simulink model "PubIfDecisionTOS_MDL"  (R2020b)
settings: configuration reference "DspaceConfig" (kept outside this file)
PostLoadFcn:
  | if any(exist('dsrtsu_mdlpostloadfcn', 'file') ~= 0), dsrtsu_mdlpostloadfcn('Execute', bdroot); end
InitFcn:
  | , if any(exist('dsmpb_private', 'file') ~= 0), dsmpb_private('dsmpb_mdlclblib', 'Init', bdroot); end,
undefined symbols (not defined in the file or in its folder): C_TOS_ACCEgoRAxletoFbumplength_m, C_TOS_ACCTargetFront_Flag, C_TOS_AEBJAPedObjDxThre_Val, C_TOS_AEBJAPedObjDyThre_Val, C_TOS_AEBJATargetSize_Val, C_TOS_AEBJAVehObjDxThre_Val, C_TOS_AEBJAVehObjDyThre_Val, C_TOS_AEBJuncPedTargetSize_Val, C_TOS_AEBLatObjDxThre_Val, C_TOS_AEBLatPedDyThre_Val, C_TOS_AEBLatTargetSize_Val, C_TOS_AEBLongTargetInEgoFront_Flag, C_TOS_axAbsGround_Parameter, C_TOS_CameraConfirmedFlag, C_TOS_CNsubjWidth, C_TOS_CurrentLaneCoreMinWidth_Val, C_TOS_CutInProb_Val_Zero, C_TOS_CutOutProb_Val_Zero, C_TOS_D2R_Val, C_TOS_DefaultValueObjectToCenterLine_dy, C_TOS_EgoCarWidth_Val, C_TOS_EgoDxRefPoint_m, C_TOS_EgoRAxletoFbumplength_m, C_TOS_HalfWidthVehicle_Con, C_TOS_HWA_CurrentLaneFlag, C_TOS_HWA_LeftLaneFlag, C_TOS_HWA_MovingDir_Vaild, C_TOS_HWA_MovState_Vaild, C_TOS_HWA_RightLaneFlag, C_TOS_LaneLineCourseErrorFront, C_TOS_LaneLineCourseErrorRear, C_TOS_MotorbikeDefaultWidth_m, C_TOS_NumberOfEffectiveTargets, C_TOS_Obj_Age_Val, C_TOS_Objdx_Constraint_Val, C_TOS_ObjectDefaultWidth_m, C_TOS_ObjInCurrentLane_Val, C_TOS_ObjInCurrentLaneValid, C_TOS_ObjInLeftLaneValid, C_TOS_ObjInRightLaneValid, C_TOS_ObjNotInCurrentLane_Val, C_TOS_ObjNotREElementType, C_TOS_ObjPredictDis_dy_ConstantVal_Zeros, C_TOS_ObjToCenterLine_ConstantVal_Zeros, C_TOS_OFMObjIDInvilad_Val, C_TOS_PIL_LatDisCons_Val_zero, C_TOS_PIL_ObjectCutInFlag_b, C_TOS_PIL_ObjectCutOutFlag_b, C_TOS_PIL_ObjLaneProb_al_Val, C_TOS_PP_ObjFusType_FC_Confirm_b, C_TOS_PP_ObjFusType_FC_FR_Confirm_b, C_TOS_PP_ObjFusType_FR_Confirm_b, C_TOS_RE_80BoolDefault_Val, C_TOS_RE_80Single181Default_Val, C_TOS_RE_80Single255Default_Val, C_TOS_RE_80Uint8Default_Val, C_TOS_RE_D2R, C_TOS_RE_D_180_Val, C_TOS_RE_InvalidObjectID_Val, C_TOS_RE_InvalidTargetChainDir_Val ... (+142)
libraries: simulink x1650, TOS_LIB x361, canfdmsglib x14
(part 4 of 69)

== system PubIfDecisionTOS_MDL/TOS_20201112/TOS_2012080320/Subsystem3 ==
  TOS_ELK : Inport
  TOS_LC : Inport  Port=2
  TOS_LCKIE : Inport  Port=3
  Bus Selector : BusSelector  OutputSignals=Object_DX,Object_DY,Object_Fus_Type,Object_Type,Object_VX
  Bus Selector1 : BusSelector  OutputSignals=Object_DX,Object_DY,Object_ExistProb,Object_Fus_Type,Object_ID,Object_Type
  Bus Selector2 : BusSelector  OutputSignals=CurrentLane_Prob,LeftLane_Prob,Object_ExistProb,Object_Fus_Type,Object_ID,Object_MovingState,Object_ObstacleProb,Object_Orientation,Object_Type,RightLane_Prob
  Bus Selector3 : BusSelector  OutputSignals=ObjectIn_Lane,Object_DX,Object_DY,Object_VX
  Bus Selector4 : BusSelector  OutputSignals=CurrentLane_Prob,LeftLane_Prob,ObjectIn_Lane,Object_ExistProb,Object_ID,Object_ObstacleProb
  Bus Selector5 : BusSelector  OutputSignals=CurrentLane_Prob,LeftLane_Prob,ObjectIn_Lane,Object_VX,RightLane_Prob
  CAN FD Pack : canfdmsglib/CAN FD Pack  CANdbFile=F:\InternalData03_ACC_AEBLog_ELK_LC_LCKie_20200927.dbc  MsgList=(none)  MsgName=TOS_ELK_1  ProtocolMode=CAN FD  MsgIDType=Standard (11-bit identifier)  MsgIdentifier=515  MsgLength=64  Remote=off  BRSSwitch=off  ApplyMinMax=off  SignalInfo={'{'ELK_CurrentLane_Prob_01','289','7','BE','unsigned','Standard','0','0.01','0','0','1.27';'ELK_CurrentLane_Prob_02','65','7','BE','unsigned','Standard','0','0.01','0','0','1.27';'ELK_CurrentLane_Prob_03','73','7','BE','unsigned','Standard','0','0.01','0','0','1.27';'ELK_CurrentLane_Prob_04','113','7','BE','unsigned','Standard','0','0.01','0','0','1.27';'ELK_CurrentLane_Prob_05','121','7','BE','unsigned','Standard','0','0.01','0','0','1.27';'ELK_CurrentLane_Prob_06','193','7','BE','unsigned','Standard','0','0.01','0','0','1.27';'ELK_CurrentLane_Prob_07','201','7','BE','unsigned','Standard','0','0.01','0','0','1.27';'ELK_CurrentLane_Prob_08','241','7','BE','unsigned','Standard','0','0.01','0','0','1.27';'ELK_LeftLane_Prob_01','281','7','BE','unsigned','Standard','0','0.01','0','0','1.27';'ELK_LeftLane_Prob_02','297','7','BE','unsigned','Standard','0','0.01','0','0','1.27';'ELK_LeftLane_Prob_03','305','7','BE','unsigned','Standard','0','0.01','0','0','1.27';'ELK_LeftLane_Prob_04','313','7','BE','unsigned','Standard','0','0.01','0','0','1.27';'ELK_LeftLane_Prob_05','321','7','BE','unsigned','Standard','0','0.01','0','0','1.27';'ELK_LeftLane_Prob_06','329','7','BE','unsigned','Standard','0','0.01','0','0','1.27';'ELK_LeftLane_Prob_07','337','7','BE','unsigned','Standard','0','0.01','0','0','1.27';'ELK_LeftLane_Prob_08','345','7','BE','unsigned','Standard','0','0.01','0','0','1.27';'ELK_Object_ExistProb_01','369','7','BE','unsigned','Standard','0','0.007875','0','0','1.0001';'ELK_Object_ExistProb_02','377','7','BE','unsigned','Standard','0','0.007875','0','0','1.0001';'ELK_Object_ExistProb_03','385','7','BE','unsigned','Standard','0','0.007875','0','0','1.0001';'ELK_Object_ExistProb_04','393','7','BE','unsigned','Standard','0','0.007875','0','0','1.0001';'ELK_Object_ExistProb_05','401','7','BE','unsigned','Standard','0','0.007875','0','0','1.0001';'ELK_Object_ExistProb_06','409','7','BE','unsigned','Standard','0','0.007875','0','0','1.0001';'ELK_Object_ExistProb_07','417','7','BE','unsigned','Standard','0','0.007875','0','0','1.0001';'ELK_Object_ExistProb_08','425','7','BE','unsigned','Standard','0','0.007875','0','0','1.0001';'ELK_Object_Fus_Type_01','452','4','BE','unsigned','Standard','0','1','0','0','15';'ELK_Object_Fus_Type_02','448','4','BE','unsigned','Standard','0','1','0','0','15';'ELK_Object_Fus_Type_03','460','4','BE','unsigned','Standard','0','1','0','0','15';'ELK_Object_Fus_Type_04','456','4','BE','unsigned','Standard','0','1','0','0','15';'ELK_Object_Fus_Type_05','468','4','BE','unsigned','Standard','0','1','0','0','15';'ELK_Object_Fus_Type_06','464','4','BE','unsigned','Standard','0','1','0','0','15';'ELK_Object_Fus_Type_07','476','4','BE','unsigned','Standard','0','1','0','0','15';'ELK_Object_Fus_Type_08','472','4','BE','unsigned','Standard','0','1','0','0','15';'ELK_Object_ID_01','1','7','BE','unsigned','Standard','0','1','0','0','127';'ELK_Object_ID_02','9','7','BE','unsigned','Standard','0','1','0','0','127';'ELK_Object_ID_03','17','7','BE','unsigned','Standard','0','1','0','0','127';'ELK_Object_ID_04','25','7','BE','unsigned','Standard','0','1','0','0','127';'ELK_Object_ID_05','33','7','BE','unsigned','Standard','0','1','0','0','127';'ELK_Object_ID_06','41','7','BE','unsigned','Standard','0','1','0','0','127';'ELK_Object_ID_07','49','7','BE','unsigned','Standard','0','1','0','0','127';'ELK_Object_ID_08','57','7','BE','unsigned','Standard','0','1','0','0','127';'ELK_Object_MovingState_01','85','3','BE','unsigned','Standard','0','1','0','0','7';'ELK_Object_MovingState_02','82','3','BE','unsigned','Standard','0','1','0','0','7';'ELK_Object_MovingState_03','93','3','BE','unsigned','Standard','0','1','0','0','7';'ELK_Object_MovingState_04','90','3','BE','unsigned','Standard','0','1','0','0','7';'ELK_Object_MovingState_05','101','3','BE','unsigned','Standard','0','1','0','0','7';'ELK_Object_MovingState_06','98','3','BE','unsigned','Standard','0','1','0','0','7';'ELK_Object_MovingState_07','109','3','BE','unsigned','Standard','0','1','0','0','7';'ELK_Object_MovingState_08','106','3','BE','unsigned','Standard','0','1','0','0','7';'ELK_Object_ObstacleProb_01','129','7','BE','unsigned','Standard','0','0.007875','0','0','1.0001';'ELK_Object_ObstacleProb_02','137','7','BE','unsigned','Standard','0','0.007875','0','0','1.0001';'ELK_Object_ObstacleProb_03','145','7','BE','unsigned','Standard','0','0.007875','0','0','1.0001';'ELK_Object_ObstacleProb_04','153','7','BE','unsigned','Standard','0','0.007875','0','0','1.0001';'ELK_Object_ObstacleProb_05','161','7','BE','unsigned','Standard','0','0.007875','0','0','1.0001';'ELK_Object_ObstacleProb_06','169','7','BE','unsigned','Standard','0','0.007875','0','0','1.0001';'ELK_Object_ObstacleProb_07','177','7','BE','unsigned','Standard','0','0.007875','0','0','1.0001';'ELK_Object_ObstacleProb_08','185','7','BE','unsigned','Standard','0','0.007875','0','0','1.0001';'ELK_Object_Orientation_01','212','4','BE','unsigned','Standard','0','1','0','0','15';'ELK_Object_Orientation_02','208','4','BE','unsigned','Standard','0','1','0','0','15';'ELK_Object_Orientation_03','220','4','BE','unsigned','Standard','0','1','0','0','15';'ELK_Object_Orientation_04','216','4','BE','unsigned','Standard','0','1','0','0','15';'ELK_Object_Orientation_05','228','4','BE','unsigned','Standard','0','1','0','0','15';'ELK_Object_Orientation_06','224','4','BE','unsigned','Standard','0','1','0','0','15';'ELK_Object_Orientation_07','236','4','BE','unsigned','Standard','0','1','0','0','15';'ELK_Object_Orientation_08','232','4','BE','unsigned','Standard','0','1','0','0','15';'ELK_Object_Type_01','252','4','BE','unsigned','Standard','0','1','0','0','15';'ELK_Object_Type_02','248','4','BE','unsigned','Standard','0','1','0','0','15';'ELK_Object_Type_03','260','4','BE','unsigned','Standard','0','1','0','0','15';'ELK_Object_Type_04','256','4','BE','unsigned','Standard','0','1','0','0','15';'ELK_Object_Type_05','268','4','BE','unsigned','Standard','0','1','0','0','15';'ELK_Object_Type_06','264','4','BE','unsigned','Standard','0','1','0','0','15';'ELK_Object_Type_07','276','4','BE','unsigned','Standard','0','1','0','0','15';'ELK_Object_Type_08','272','4','BE','unsigned','Standard','0','1','0','0','15';'ELK_RightLane_Prob_01','353','7','BE','unsigned','Standard','0','0.01','0','0','1.27';'ELK_RightLane_Prob_02','361','7','BE','unsigned','Standard','0','0.01','0','0','1.27';'ELK_RightLane_Prob_03','433','7','BE','unsigned','Standard','0','0.01','0','0','1.27';'ELK_RightLane_Prob_04','441','7','BE','unsigned','Standard','0','0.01','0','0','1.27';'ELK_RightLane_Prob_05','481','7','BE','unsigned','Standard','0','0.01','0','0','1.27';'ELK_RightLane_Prob_06','489','7','BE','unsigned','Standard','0','0.01','0','0','1.27';'ELK_RightLane_Prob_07','497','7','BE','unsigned','Standard','0','0.01','0','0','1.27'}
      settings: SourceProductBaseCode=VN  DataFormat=CANdb specified signals
  CAN FD Pack1 : canfdmsglib/CAN FD Pack  CANdbFile=F:\InternalData03_ACC_AEBLog_ELK_LC_LCKie_20200927.dbc  MsgList=(none)  MsgName=TOS_ELK_2  ProtocolMode=CAN FD  MsgIDType=Standard (11-bit identifier)  MsgIdentifier=516  MsgLength=64  Remote=off  BRSSwitch=off  ApplyMinMax=off  SignalInfo={'{'ELK_ObjectIn_Lane_01','132','4','BE','unsigned','Standard','0','1','0','0','15';'ELK_ObjectIn_Lane_02','128','4','BE','unsigned','Standard','0','1','0','0','15';'ELK_ObjectIn_Lane_03','140','4','BE','unsigned','Standard','0','1','0','0','15';'ELK_ObjectIn_Lane_04','136','4','BE','unsigned','Standard','0','1','0','0','15';'ELK_ObjectIn_Lane_05','148','4','BE','unsigned','Standard','0','1','0','0','15';'ELK_ObjectIn_Lane_06','144','4','BE','unsigned','Standard','0','1','0','0','15';'ELK_ObjectIn_Lane_07','156','4','BE','unsigned','Standard','0','1','0','0','15';'ELK_ObjectIn_Lane_08','152','4','BE','unsigned','Standard','0','1','0','0','15';'ELK_Object_DX_01','8','16','BE','signed','Standard','0','0.01','0','-327.68','327.67';'ELK_Object_DX_02','24','16','BE','signed','Standard','0','0.01','0','-327.68','327.67';'ELK_Object_DX_03','40','16','BE','signed','Standard','0','0.01','0','-327.68','327.67';'ELK_Object_DX_04','56','16','BE','signed','Standard','0','0.01','0','-327.68','327.67';'ELK_Object_DX_05','72','16','BE','signed','Standard','0','0.01','0','-327.68','327.67';'ELK_Object_DX_06','88','16','BE','signed','Standard','0','0.01','0','-327.68','327.67';'ELK_Object_DX_07','104','16','BE','signed','Standard','0','0.01','0','-327.68','327.67';'ELK_Object_DX_08','120','16','BE','signed','Standard','0','0.01','0','-327.68','327.67';'ELK_Object_DY_01','168','16','BE','signed','Standard','0','0.01','0','-327.68','327.67';'ELK_Object_DY_02','184','16','BE','signed','Standard','0','0.01','0','-327.68','327.67';'ELK_Object_DY_03','200','16','BE','signed','Standard','0','0.01','0','-327.68','327.67';'ELK_Object_DY_04','216','16','BE','signed','Standard','0','0.01','0','-327.68','327.67';'ELK_Object_DY_05','232','16','BE','signed','Standard','0','0.01','0','-327.68','327.67';'ELK_Object_DY_06','248','16','BE','signed','Standard','0','0.01','0','-327.68','327.67';'ELK_Object_DY_07','264','16','BE','signed','Standard','0','0.01','0','-327.68','327.67';'ELK_Object_DY_08','280','16','BE','signed','Standard','0','0.01','0','-327.68','327.67';'ELK_Object_VX_01','332','12','BE','signed','Standard','0','0.1','0','-204.8','204.7';'ELK_Object_VX_02','348','12','BE','signed','Standard','0','0.1','0','-204.8','204.7';'ELK_Object_VX_03','364','12','BE','signed','Standard','0','0.1','0','-204.8','204.7';'ELK_Object_VX_04','380','12','BE','signed','Standard','0','0.1','0','-204.8','204.7';'ELK_Object_VX_05','396','12','BE','signed','Standard','0','0.1','0','-204.8','204.7';'ELK_Object_VX_06','412','12','BE','signed','Standard','0','0.1','0','-204.8','204.7';'ELK_Object_VX_07','428','12','BE','signed','Standard','0','0.1','0','-204.8','204.7'}
      settings: SourceProductBaseCode=VN  DataFormat=CANdb specified signals
  CAN FD Pack2 : canfdmsglib/CAN FD Pack  CANdbFile=F:\InternalData03_ACC_AEBLog_ELK_LC_LCKie_20200927.dbc  MsgList=(none)  MsgName=TOS_LC_1  ProtocolMode=CAN FD  MsgIDType=Standard (11-bit identifier)  MsgIdentifier=519  MsgLength=64  Remote=off  BRSSwitch=off  ApplyMinMax=off  SignalInfo={'{'LC_Object_DX_01','12','12','BE','signed','Standard','0','0.1','0','-204.8','204.7';'LC_Object_DX_02','28','12','BE','signed','Standard','0','0.1','0','-204.8','204.7';'LC_Object_DX_03','44','12','BE','signed','Standard','0','0.1','0','-204.8','204.7';'LC_Object_DX_04','60','12','BE','signed','Standard','0','0.1','0','-204.8','204.7';'LC_Object_DX_05','76','12','BE','signed','Standard','0','0.1','0','-204.8','204.7';'LC_Object_DX_06','92','12','BE','signed','Standard','0','0.1','0','-204.8','204.7';'LC_Object_DX_07','108','12','BE','signed','Standard','0','0.1','0','-204.8','204.7';'LC_Object_DX_08','124','12','BE','signed','Standard','0','0.1','0','-204.8','204.7';'LC_Object_DX_09','140','12','BE','signed','Standard','0','0.1','0','-204.8','204.7';'LC_Object_DX_10','156','12','BE','signed','Standard','0','0.1','0','-204.8','204.7';'LC_Object_DX_11','172','12','BE','signed','Standard','0','0.1','0','-204.8','204.7';'LC_Object_DY_01','188','12','BE','signed','Standard','0','0.1','0','-204.8','204.7';'LC_Object_DY_02','204','12','BE','signed','Standard','0','0.1','0','-204.8','204.7';'LC_Object_DY_03','220','12','BE','signed','Standard','0','0.1','0','-204.8','204.7';'LC_Object_DY_04','236','12','BE','signed','Standard','0','0.1','0','-204.8','204.7';'LC_Object_DY_05','252','12','BE','signed','Standard','0','0.1','0','-204.8','204.7';'LC_Object_DY_06','268','12','BE','signed','Standard','0','0.1','0','-204.8','204.7';'LC_Object_DY_07','284','12','BE','signed','Standard','0','0.1','0','-204.8','204.7';'LC_Object_DY_08','300','12','BE','signed','Standard','0','0.1','0','-204.8','204.7';'LC_Object_DY_09','316','12','BE','signed','Standard','0','0.1','0','-204.8','204.7';'LC_Object_DY_10','332','12','BE','signed','Standard','0','0.1','0','-204.8','204.7';'LC_Object_DY_11','348','12','BE','signed','Standard','0','0.1','0','-204.8','204.7';'LC_Object_Fus_Type_01','8','4','BE','unsigned','Standard','0','1','0','0','15';'LC_Object_Fus_Type_02','24','4','BE','unsigned','Standard','0','1','0','0','15';'LC_Object_Fus_Type_03','40','4','BE','unsigned','Standard','0','1','0','0','15';'LC_Object_Fus_Type_04','56','4','BE','unsigned','Standard','0','1','0','0','15';'LC_Object_Fus_Type_05','72','4','BE','unsigned','Standard','0','1','0','0','15';'LC_Object_Fus_Type_06','88','4','BE','unsigned','Standard','0','1','0','0','15';'LC_Object_Fus_Type_07','104','4','BE','unsigned','Standard','0','1','0','0','15';'LC_Object_Fus_Type_08','120','4','BE','unsigned','Standard','0','1','0','0','15';'LC_Object_Fus_Type_09','136','4','BE','unsigned','Standard','0','1','0','0','15';'LC_Object_Fus_Type_10','152','4','BE','unsigned','Standard','0','1','0','0','15';'LC_Object_Fus_Type_11','168','4','BE','unsigned','Standard','0','1','0','0','15';'LC_Object_Type_01','184','4','BE','unsigned','Standard','0','1','0','0','15';'LC_Object_Type_02','200','4','BE','unsigned','Standard','0','1','0','0','15';'LC_Object_Type_03','216','4','BE','unsigned','Standard','0','1','0','0','15';'LC_Object_Type_04','232','4','BE','unsigned','Standard','0','1','0','0','15';'LC_Object_Type_05','248','4','BE','unsigned','Standard','0','1','0','0','15';'LC_Object_Type_06','264','4','BE','unsigned','Standard','0','1','0','0','15';'LC_Object_Type_07','280','4','BE','unsigned','Standard','0','1','0','0','15';'LC_Object_Type_08','296','4','BE','unsigned','Standard','0','1','0','0','15';'LC_Object_Type_09','312','4','BE','unsigned','Standard','0','1','0','0','15';'LC_Object_Type_10','328','4','BE','unsigned','Standard','0','1','0','0','15';'LC_Object_Type_11','344','4','BE','unsigned','Standard','0','1','0','0','15';'LC_Object_VX_01','384','12','BE','signed','Standard','0','0.1','0','-204.8','204.7';'LC_Object_VX_02','404','12','BE','signed','Standard','0','0.1','0','-204.8','204.7';'LC_Object_VX_03','408','12','BE','signed','Standard','0','0.1','0','-204.8','204.7';'LC_Object_VX_04','428','12','BE','signed','Standard','0','0.1','0','-204.8','204.7';'LC_Object_VX_05','432','12','BE','signed','Standard','0','0.1','0','-204.8','204.7';'LC_Object_VX_06','452','12','BE','signed','Standard','0','0.1','0','-204.8','204.7';'LC_Object_VX_07','456','12','BE','signed','Standard','0','0.1','0','-204.8','204.7';'LC_Object_VX_08','476','12','BE','signed','Standard','0','0.1','0','-204.8','204.7';'LC_Object_VX_09','480','12','BE','signed','Standard','0','0.1','0','-204.8','204.7';'LC_Object_VX_10','500','12','BE','signed','Standard','0','0.1','0','-204.8','204.7'}
      settings: SourceProductBaseCode=VN  DataFormat=CANdb specified signals
  CAN FD Pack3 : canfdmsglib/CAN FD Pack  CANdbFile=F:\InternalData03_ACC_AEBLog_ELK_LC_LCKie_20200927.dbc  MsgList=(none)  MsgName=TOS_LC_2  ProtocolMode=CAN FD  MsgIDType=Standard (11-bit identifier)  MsgIdentifier=520  MsgLength=64  Remote=off  BRSSwitch=off  ApplyMinMax=off  SignalInfo={'{'LC_CurrentLane_Prob_01','265','7','BE','unsigned','Standard','0','0.01','0','0','1.27';'LC_CurrentLane_Prob_02','273','7','BE','unsigned','Standard','0','0.01','0','0','1.27';'LC_CurrentLane_Prob_03','281','7','BE','unsigned','Standard','0','0.01','0','0','1.27';'LC_CurrentLane_Prob_04','289','7','BE','unsigned','Standard','0','0.01','0','0','1.27';'LC_CurrentLane_Prob_05','297','7','BE','unsigned','Standard','0','0.01','0','0','1.27';'LC_CurrentLane_Prob_06','305','7','BE','unsigned','Standard','0','0.01','0','0','1.27';'LC_CurrentLane_Prob_07','313','7','BE','unsigned','Standard','0','0.01','0','0','1.27';'LC_CurrentLane_Prob_08','321','7','BE','unsigned','Standard','0','0.01','0','0','1.27';'LC_CurrentLane_Prob_09','329','7','BE','unsigned','Standard','0','0.01','0','0','1.27';'LC_CurrentLane_Prob_10','337','7','BE','unsigned','Standard','0','0.01','0','0','1.27';'LC_CurrentLane_Prob_11','345','7','BE','unsigned','Standard','0','0.01','0','0','1.27';'LC_LeftLane_Prob_01','353','7','BE','unsigned','Standard','0','0.01','0','0','1.27';'LC_LeftLane_Prob_02','361','7','BE','unsigned','Standard','0','0.01','0','0','1.27';'LC_LeftLane_Prob_03','369','7','BE','unsigned','Standard','0','0.01','0','0','1.27';'LC_LeftLane_Prob_04','377','7','BE','unsigned','Standard','0','0.01','0','0','1.27';'LC_LeftLane_Prob_05','385','7','BE','unsigned','Standard','0','0.01','0','0','1.27';'LC_LeftLane_Prob_06','393','7','BE','unsigned','Standard','0','0.01','0','0','1.27';'LC_LeftLane_Prob_07','401','7','BE','unsigned','Standard','0','0.01','0','0','1.27';'LC_LeftLane_Prob_08','409','7','BE','unsigned','Standard','0','0.01','0','0','1.27';'LC_LeftLane_Prob_09','417','7','BE','unsigned','Standard','0','0.01','0','0','1.27';'LC_LeftLane_Prob_10','425','7','BE','unsigned','Standard','0','0.01','0','0','1.27';'LC_LeftLane_Prob_11','433','7','BE','unsigned','Standard','0','0.01','0','0','1.27';'LC_ObjectIn_Lane_01','444','4','BE','unsigned','Standard','0','1','0','0','15';'LC_ObjectIn_Lane_02','440','4','BE','unsigned','Standard','0','1','0','0','15';'LC_ObjectIn_Lane_03','452','4','BE','unsigned','Standard','0','1','0','0','15';'LC_ObjectIn_Lane_04','448','4','BE','unsigned','Standard','0','1','0','0','15';'LC_ObjectIn_Lane_05','460','4','BE','unsigned','Standard','0','1','0','0','15';'LC_ObjectIn_Lane_06','456','4','BE','unsigned','Standard','0','1','0','0','15';'LC_ObjectIn_Lane_07','468','4','BE','unsigned','Standard','0','1','0','0','15';'LC_ObjectIn_Lane_08','464','4','BE','unsigned','Standard','0','1','0','0','15';'LC_ObjectIn_Lane_09','476','4','BE','unsigned','Standard','0','1','0','0','15';'LC_ObjectIn_Lane_10','472','4','BE','unsigned','Standard','0','1','0','0','15';'LC_ObjectIn_Lane_11','484','4','BE','unsigned','Standard','0','1','0','0','15';'LC_Object_ExistProb_01','1','7','BE','unsigned','Standard','0','0.007875','0','0','1.0001';'LC_Object_ExistProb_02','9','7','BE','unsigned','Standard','0','0.007875','0','0','1.0001';'LC_Object_ExistProb_03','17','7','BE','unsigned','Standard','0','0.007875','0','0','1.0001';'LC_Object_ExistProb_04','25','7','BE','unsigned','Standard','0','0.007875','0','0','1.0001';'LC_Object_ExistProb_05','33','7','BE','unsigned','Standard','0','0.007875','0','0','1.0001';'LC_Object_ExistProb_06','41','7','BE','unsigned','Standard','0','0.007875','0','0','1.0001';'LC_Object_ExistProb_07','49','7','BE','unsigned','Standard','0','0.007875','0','0','1.0001';'LC_Object_ExistProb_08','57','7','BE','unsigned','Standard','0','0.007875','0','0','1.0001';'LC_Object_ExistProb_09','65','7','BE','unsigned','Standard','0','0.007875','0','0','1.0001';'LC_Object_ExistProb_10','73','7','BE','unsigned','Standard','0','0.007875','0','0','1.0001';'LC_Object_ExistProb_11','81','7','BE','unsigned','Standard','0','0.007875','0','0','1.0001';'LC_Object_ID_01','89','7','BE','unsigned','Standard','0','1','0','0','127';'LC_Object_ID_02','97','7','BE','unsigned','Standard','0','1','0','0','127';'LC_Object_ID_03','105','7','BE','unsigned','Standard','0','1','0','0','127';'LC_Object_ID_04','113','7','BE','unsigned','Standard','0','1','0','0','127';'LC_Object_ID_05','121','7','BE','unsigned','Standard','0','1','0','0','127';'LC_Object_ID_06','129','7','BE','unsigned','Standard','0','1','0','0','127';'LC_Object_ID_07','137','7','BE','unsigned','Standard','0','1','0','0','127';'LC_Object_ID_08','145','7','BE','unsigned','Standard','0','1','0','0','127';'LC_Object_ID_09','153','7','BE','unsigned','Standard','0','1','0','0','127';'LC_Object_ID_10','161','7','BE','unsigned','Standard','0','1','0','0','127';'LC_Object_ID_11','169','7','BE','unsigned','Standard','0','1','0','0','127';'LC_Object_ObstacleProb_01','177','7','BE','unsigned','Standard','0','0.007875','0','0','1.0001';'LC_Object_ObstacleProb_02','185','7','BE','unsigned','Standard','0','0.007875','0','0','1.0001';'LC_Object_ObstacleProb_03','193','7','BE','unsigned','Standard','0','0.007875','0','0','1.0001';'LC_Object_ObstacleProb_04','201','7','BE','unsigned','Standard','0','0.007875','0','0','1.0001';'LC_Object_ObstacleProb_05','209','7','BE','unsigned','Standard','0','0.007875','0','0','1.0001';'LC_Object_ObstacleProb_06','217','7','BE','unsigned','Standard','0','0.007875','0','0','1.0001';'LC_Object_ObstacleProb_07','225','7','BE','unsigned','Standard','0','0.007875','0','0','1.0001';'LC_Object_ObstacleProb_08','233','7','BE','unsigned','Standard','0','0.007875','0','0','1.0001';'LC_Object_ObstacleProb_09','241','7','BE','unsigned','Standard','0','0.007875','0','0','1.0001';'LC_Object_ObstacleProb_10','249','7','BE','unsigned','Standard','0','0.007875','0','0','1.0001'}
      settings: SourceProductBaseCode=VN  DataFormat=CANdb specified signals
  CAN FD Pack4 : canfdmsglib/CAN FD Pack  CANdbFile=F:\InternalData03_ACC_AEBLog_ELK_LC_LCKie_20200927.dbc  MsgList=(none)  MsgName=TOS_LCKie_1  ProtocolMode=CAN FD  MsgIDType=Standard (11-bit identifier)  MsgIdentifier=517  MsgLength=64  Remote=off  BRSSwitch=off  ApplyMinMax=off  SignalInfo={'{'LCKIE_Object_DX_01','8','16','BE','signed','Standard','0','0.01','0','-327.68','327.67';'LCKIE_Object_DX_02','24','16','BE','signed','Standard','0','0.01','0','-327.68','327.67';'LCKIE_Object_DX_03','40','16','BE','signed','Standard','0','0.01','0','-327.68','327.67';'LCKIE_Object_DX_04','56','16','BE','signed','Standard','0','0.01','0','-327.68','327.67';'LCKIE_Object_DX_05','72','16','BE','signed','Standard','0','0.01','0','-327.68','327.67';'LCKIE_Object_DX_06','88','16','BE','signed','Standard','0','0.01','0','-327.68','327.67';'LCKIE_Object_DX_07','104','16','BE','signed','Standard','0','0.01','0','-327.68','327.67';'LCKIE_Object_DX_08','120','16','BE','signed','Standard','0','0.01','0','-327.68','327.67';'LCKIE_Object_DX_09','136','16','BE','signed','Standard','0','0.01','0','-327.68','327.67';'LCKIE_Object_DY_01','152','16','BE','signed','Standard','0','0.01','0','-327.68','327.67';'LCKIE_Object_DY_02','168','16','BE','signed','Standard','0','0.01','0','-327.68','327.67';'LCKIE_Object_DY_03','312','16','BE','signed','Standard','0','0.01','0','-327.68','327.67';'LCKIE_Object_DY_04','360','16','BE','signed','Standard','0','0.01','0','-327.68','327.67';'LCKIE_Object_DY_05','376','16','BE','signed','Standard','0','0.01','0','-327.68','327.67';'LCKIE_Object_DY_06','392','16','BE','signed','Standard','0','0.01','0','-327.68','327.67';'LCKIE_Object_DY_07','408','16','BE','signed','Standard','0','0.01','0','-327.68','327.67';'LCKIE_Object_DY_08','424','16','BE','signed','Standard','0','0.01','0','-327.68','327.67';'LCKIE_Object_DY_09','440','16','BE','signed','Standard','0','0.01','0','-327.68','327.67';'LCKIE_Object_ExistProb_01','297','7','BE','unsigned','Standard','0','0.007875','0','0','1.0001';'LCKIE_Object_ExistProb_02','449','7','BE','unsigned','Standard','0','0.007875','0','0','1.0001';'LCKIE_Object_ExistProb_03','457','7','BE','unsigned','Standard','0','0.007875','0','0','1.0001';'LCKIE_Object_ExistProb_04','465','7','BE','unsigned','Standard','0','0.007875','0','0','1.0001';'LCKIE_Object_ExistProb_05','473','7','BE','unsigned','Standard','0','0.007875','0','0','1.0001';'LCKIE_Object_ExistProb_06','481','7','BE','unsigned','Standard','0','0.007875','0','0','1.0001';'LCKIE_Object_ExistProb_07','489','7','BE','unsigned','Standard','0','0.007875','0','0','1.0001';'LCKIE_Object_ExistProb_08','497','7','BE','unsigned','Standard','0','0.007875','0','0','1.0001';'LCKIE_Object_ExistProb_09','505','7','BE','unsigned','Standard','0','0.007875','0','0','1.0001';'LCKIE_Object_Fus_Type_01','180','4','BE','unsigned','Standard','0','1','0','0','15';'LCKIE_Object_Fus_Type_02','176','4','BE','unsigned','Standard','0','1','0','0','15';'LCKIE_Object_Fus_Type_03','188','4','BE','unsigned','Standard','0','1','0','0','15';'LCKIE_Object_Fus_Type_04','184','4','BE','unsigned','Standard','0','1','0','0','15';'LCKIE_Object_Fus_Type_05','196','4','BE','unsigned','Standard','0','1','0','0','15';'LCKIE_Object_Fus_Type_06','192','4','BE','unsigned','Standard','0','1','0','0','15';'LCKIE_Object_Fus_Type_07','204','4','BE','unsigned','Standard','0','1','0','0','15';'LCKIE_Object_Fus_Type_08','200','4','BE','unsigned','Standard','0','1','0','0','15';'LCKIE_Object_Fus_Type_09','212','4','BE','unsigned','Standard','0','1','0','0','15';'LCKIE_Object_ID_01','225','7','BE','unsigned','Standard','0','1','0','0','127';'LCKIE_Object_ID_02','233','7','BE','unsigned','Standard','0','1','0','0','127';'LCKIE_Object_ID_03','241','7','BE','unsigned','Standard','0','1','0','0','127';'LCKIE_Object_ID_04','249','7','BE','unsigned','Standard','0','1','0','0','127';'LCKIE_Object_ID_05','257','7','BE','unsigned','Standard','0','1','0','0','127';'LCKIE_Object_ID_06','265','7','BE','unsigned','Standard','0','1','0','0','127';'LCKIE_Object_ID_07','273','7','BE','unsigned','Standard','0','1','0','0','127';'LCKIE_Object_ID_08','281','7','BE','unsigned','Standard','0','1','0','0','127';'LCKIE_Object_ID_09','289','7','BE','unsigned','Standard','0','1','0','0','127';'LCKIE_Object_Type_01','216','4','BE','unsigned','Standard','0','1','0','0','15';'LCKIE_Object_Type_02','324','4','BE','unsigned','Standard','0','1','0','0','15';'LCKIE_Object_Type_03','320','4','BE','unsigned','Standard','0','1','0','0','15';'LCKIE_Object_Type_04','332','4','BE','unsigned','Standard','0','1','0','0','15';'LCKIE_Object_Type_05','328','4','BE','unsigned','Standard','0','1','0','0','15';'LCKIE_Object_Type_06','340','4','BE','unsigned','Standard','0','1','0','0','15';'LCKIE_Object_Type_07','336','4','BE','unsigned','Standard','0','1','0','0','15';'LCKIE_Object_Type_08','348','4','BE','unsigned','Standard','0','1','0','0','15'}
      settings: SourceProductBaseCode=VN  DataFormat=CANdb specified signals
  CAN FD Pack5 : canfdmsglib/CAN FD Pack  CANdbFile=F:\InternalData03_ACC_AEBLog_ELK_LC_LCKie_20200927.dbc  MsgList=(none)  MsgName=TOS_LCKie_2  ProtocolMode=CAN FD  MsgIDType=Standard (11-bit identifier)  MsgIdentifier=518  MsgLength=64  Remote=off  BRSSwitch=off  ApplyMinMax=off  SignalInfo={'{'LCKIE_CurrentLane_Prob_01','1','7','BE','unsigned','Standard','0','0.01','0','0','1.27';'LCKIE_CurrentLane_Prob_02','9','7','BE','unsigned','Standard','0','0.01','0','0','1.27';'LCKIE_CurrentLane_Prob_03','17','7','BE','unsigned','Standard','0','0.01','0','0','1.27';'LCKIE_CurrentLane_Prob_04','25','7','BE','unsigned','Standard','0','0.01','0','0','1.27';'LCKIE_CurrentLane_Prob_05','33','7','BE','unsigned','Standard','0','0.01','0','0','1.27';'LCKIE_CurrentLane_Prob_06','41','7','BE','unsigned','Standard','0','0.01','0','0','1.27';'LCKIE_CurrentLane_Prob_07','49','7','BE','unsigned','Standard','0','0.01','0','0','1.27';'LCKIE_CurrentLane_Prob_08','57','7','BE','unsigned','Standard','0','0.01','0','0','1.27';'LCKIE_CurrentLane_Prob_09','65','7','BE','unsigned','Standard','0','0.01','0','0','1.27';'LCKIE_LeftLane_Prob_01','73','7','BE','unsigned','Standard','0','0.01','0','0','1.27';'LCKIE_LeftLane_Prob_02','81','7','BE','unsigned','Standard','0','0.01','0','0','1.27';'LCKIE_LeftLane_Prob_03','89','7','BE','unsigned','Standard','0','0.01','0','0','1.27';'LCKIE_LeftLane_Prob_04','97','7','BE','unsigned','Standard','0','0.01','0','0','1.27';'LCKIE_LeftLane_Prob_05','105','7','BE','unsigned','Standard','0','0.01','0','0','1.27';'LCKIE_LeftLane_Prob_06','113','7','BE','unsigned','Standard','0','0.01','0','0','1.27';'LCKIE_LeftLane_Prob_07','121','7','BE','unsigned','Standard','0','0.01','0','0','1.27';'LCKIE_LeftLane_Prob_08','129','7','BE','unsigned','Standard','0','0.01','0','0','1.27';'LCKIE_LeftLane_Prob_09','137','7','BE','unsigned','Standard','0','0.01','0','0','1.27';'LCKIE_ObjectIn_Lane_01','184','4','BE','unsigned','Standard','0','1','0','0','15';'LCKIE_ObjectIn_Lane_02','200','4','BE','unsigned','Standard','0','1','0','0','15';'LCKIE_ObjectIn_Lane_03','216','4','BE','unsigned','Standard','0','1','0','0','15';'LCKIE_ObjectIn_Lane_04','232','4','BE','unsigned','Standard','0','1','0','0','15';'LCKIE_ObjectIn_Lane_05','248','4','BE','unsigned','Standard','0','1','0','0','15';'LCKIE_ObjectIn_Lane_06','264','4','BE','unsigned','Standard','0','1','0','0','15';'LCKIE_ObjectIn_Lane_07','280','4','BE','unsigned','Standard','0','1','0','0','15';'LCKIE_ObjectIn_Lane_08','296','4','BE','unsigned','Standard','0','1','0','0','15';'LCKIE_ObjectIn_Lane_09','312','4','BE','unsigned','Standard','0','1','0','0','15';'LCKIE_Object_VX_01','188','12','BE','signed','Standard','0','0.1','0','-204.8','204.7';'LCKIE_Object_VX_02','204','12','BE','signed','Standard','0','0.1','0','-204.8','204.7';'LCKIE_Object_VX_03','220','12','BE','signed','Standard','0','0.1','0','-204.8','204.7';'LCKIE_Object_VX_04','236','12','BE','signed','Standard','0','0.1','0','-204.8','204.7';'LCKIE_Object_VX_05','252','12','BE','signed','Standard','0','0.1','0','-204.8','204.7';'LCKIE_Object_VX_06','268','12','BE','signed','Standard','0','0.1','0','-204.8','204.7';'LCKIE_Object_VX_07','284','12','BE','signed','Standard','0','0.1','0','-204.8','204.7';'LCKIE_Object_VX_08','300','12','BE','signed','Standard','0','0.1','0','-204.8','204.7';'LCKIE_Object_VX_09','316','12','BE','signed','Standard','0','0.1','0','-204.8','204.7';'LCKIE_RightLane_Prob_01','145','7','BE','unsigned','Standard','0','0.01','0','0','1.27';'LCKIE_RightLane_Prob_02','153','7','BE','unsigned','Standard','0','0.01','0','0','1.27';'LCKIE_RightLane_Prob_03','161','7','BE','unsigned','Standard','0','0.01','0','0','1.27';'LCKIE_RightLane_Prob_04','169','7','BE','unsigned','Standard','0','0.01','0','0','1.27';'LCKIE_RightLane_Prob_05','321','7','BE','unsigned','Standard','0','0.01','0','0','1.27';'LCKIE_RightLane_Prob_06','329','7','BE','unsigned','Standard','0','0.01','0','0','1.27';'LCKIE_RightLane_Prob_07','337','7','BE','unsigned','Standard','0','0.01','0','0','1.27';'LCKIE_RightLane_Prob_08','345','7','BE','unsigned','Standard','0','0.01','0','0','1.27'}
      settings: SourceProductBaseCode=VN  DataFormat=CANdb specified signals
  Demux{,1..13} (14 alike) : Demux  Outputs=8
  Demux{14..24} (11 alike) : Demux  Outputs=11
  Demux{25..35} (11 alike) : Demux  Outputs=9
  TOS_ELK1_Msg : Outport
  TOS_ELK2_Msg : Outport  Port=2
  TOS_LC1_Msg : Outport  Port=3
  TOS_LC2_Msg : Outport  Port=4
  TOS_LCKie1_Msg : Outport  Port=5
  TOS_LCKie2_Msg : Outport  Port=6
  wires:
  TOS_ELK/1 -> Bus Selector3/1, Bus Selector2/1
  TOS_LC/1 -> Bus Selector4/1, Bus Selector/1
  CAN FD Pack/1 -> TOS_ELK1_Msg/1
  Bus Selector2/1 -> Demux/1  "<CurrentLane_Prob>"
  Demux/1 -> CAN FD Pack/1
  Demux/2 -> CAN FD Pack/2
  Demux/3 -> CAN FD Pack/3
  Demux/4 -> CAN FD Pack/4
  Demux/5 -> CAN FD Pack/5
  Demux/6 -> CAN FD Pack/6
  Demux/7 -> CAN FD Pack/7
  Demux/8 -> CAN FD Pack/8
  Demux1/8 -> CAN FD Pack/16
  Demux1/7 -> CAN FD Pack/15
  Demux1/6 -> CAN FD Pack/14
  Demux1/5 -> CAN FD Pack/13
  Demux1/4 -> CAN FD Pack/12
  Demux1/3 -> CAN FD Pack/11
  Demux1/2 -> CAN FD Pack/10
  Demux1/1 -> CAN FD Pack/9
  Bus Selector2/2 -> Demux1/1  "<LeftLane_Prob>"
  Bus Selector2/4 -> Demux3/1  "<Object_Fus_Type>"
  Demux3/1 -> CAN FD Pack/25
  Demux3/2 -> CAN FD Pack/26
  Demux3/3 -> CAN FD Pack/27
  Demux3/4 -> CAN FD Pack/28
  Demux3/5 -> CAN FD Pack/29
  Demux3/6 -> CAN FD Pack/30
  Demux3/7 -> CAN FD Pack/31
  Demux3/8 -> CAN FD Pack/32
  Demux2/8 -> CAN FD Pack/24
  Demux2/7 -> CAN FD Pack/23
  Demux2/6 -> CAN FD Pack/22
  Demux2/5 -> CAN FD Pack/21
  Demux2/4 -> CAN FD Pack/20
  Demux2/3 -> CAN FD Pack/19
  Demux2/2 -> CAN FD Pack/18
  Demux2/1 -> CAN FD Pack/17
  Bus Selector2/3 -> Demux2/1  "<Object_ExistProb>"
  Bus Selector2/7 -> Demux6/1  "<Object_ObstacleProb>"
  Demux6/1 -> CAN FD Pack/49
  Demux6/2 -> CAN FD Pack/50
  Demux6/3 -> CAN FD Pack/51
  Demux6/4 -> CAN FD Pack/52
  Demux6/5 -> CAN FD Pack/53
  Demux6/6 -> CAN FD Pack/54
  Demux6/7 -> CAN FD Pack/55
  Demux6/8 -> CAN FD Pack/56
  Demux7/8 -> CAN FD Pack/64
  Demux7/7 -> CAN FD Pack/63
  Demux7/6 -> CAN FD Pack/62
  Demux7/5 -> CAN FD Pack/61
  Demux7/4 -> CAN FD Pack/60
  Demux7/3 -> CAN FD Pack/59
  Demux7/2 -> CAN FD Pack/58
  Demux7/1 -> CAN FD Pack/57
  Bus Selector2/8 -> Demux7/1  "<Object_Orientation>"
  Bus Selector2/6 -> Demux5/1  "<Object_MovingState>"
  Demux5/1 -> CAN FD Pack/41
  Demux5/2 -> CAN FD Pack/42
  Demux5/3 -> CAN FD Pack/43
  Demux5/4 -> CAN FD Pack/44
  Demux5/5 -> CAN FD Pack/45
  Demux5/6 -> CAN FD Pack/46
  Demux5/7 -> CAN FD Pack/47
  Demux5/8 -> CAN FD Pack/48
  Demux4/8 -> CAN FD Pack/40
  Demux4/7 -> CAN FD Pack/39
  Demux4/6 -> CAN FD Pack/38
  Demux4/5 -> CAN FD Pack/37
  Demux4/4 -> CAN FD Pack/36
  Demux4/3 -> CAN FD Pack/35
  Demux4/2 -> CAN FD Pack/34
  Demux4/1 -> CAN FD Pack/33
  Bus Selector2/5 -> Demux4/1  "<Object_ID>"
  Bus Selector2/10 -> Demux9/1  "<RightLane_Prob>"
  Demux9/1 -> CAN FD Pack/73
  Demux9/2 -> CAN FD Pack/74
  Demux9/3 -> CAN FD Pack/75
  Demux9/4 -> CAN FD Pack/76
  Demux9/5 -> CAN FD Pack/77
  Demux9/6 -> CAN FD Pack/78
  Demux9/7 -> CAN FD Pack/79
  Demux9/8 -> CAN FD Pack/80
  Demux8/8 -> CAN FD Pack/72
  Demux8/7 -> CAN FD Pack/71
  Demux8/6 -> CAN FD Pack/70
  Demux8/5 -> CAN FD Pack/69
  Demux8/4 -> CAN FD Pack/68
  Demux8/3 -> CAN FD Pack/67
  Demux8/2 -> CAN FD Pack/66
  Demux8/1 -> CAN FD Pack/65
  Bus Selector2/9 -> Demux8/1  "<Object_Type>"
  Bus Selector3/1 -> Demux10/1  "<ObjectIn_Lane>"
  Demux10/8 -> CAN FD Pack1/8
  Demux10/7 -> CAN FD Pack1/7
  Demux10/6 -> CAN FD Pack1/6
  Demux10/5 -> CAN FD Pack1/5
  Demux10/4 -> CAN FD Pack1/4
  Demux10/3 -> CAN FD Pack1/3
  Demux10/2 -> CAN FD Pack1/2
  Demux10/1 -> CAN FD Pack1/1
  Demux11/1 -> CAN FD Pack1/9
  Demux11/2 -> CAN FD Pack1/10
  Demux11/3 -> CAN FD Pack1/11
  Demux11/4 -> CAN FD Pack1/12
  Demux11/5 -> CAN FD Pack1/13
  Demux11/6 -> CAN FD Pack1/14
  Demux11/7 -> CAN FD Pack1/15
  Demux11/8 -> CAN FD Pack1/16
  Bus Selector3/2 -> Demux11/1  "<Object_DX>"
  Bus Selector3/3 -> Demux12/1  "<Object_DY>"
  Demux12/1 -> CAN FD Pack1/17
  Demux12/2 -> CAN FD Pack1/18
  Demux12/3 -> CAN FD Pack1/19
  Demux12/4 -> CAN FD Pack1/20
  Demux12/5 -> CAN FD Pack1/21
  Demux12/6 -> CAN FD Pack1/22
  Demux12/7 -> CAN FD Pack1/23
  Demux12/8 -> CAN FD Pack1/24
  Demux13/1 -> CAN FD Pack1/25
  Demux13/2 -> CAN FD Pack1/26
  Demux13/3 -> CAN FD Pack1/27
  Demux13/4 -> CAN FD Pack1/28
  Demux13/5 -> CAN FD Pack1/29
  Demux13/6 -> CAN FD Pack1/30
  Demux13/7 -> CAN FD Pack1/31
  Demux13/8 -> CAN FD Pack1/32
  Bus Selector3/4 -> Demux13/1  "<Object_VX>"
  CAN FD Pack1/1 -> TOS_ELK2_Msg/1
  Bus Selector/1 -> Demux14/1  "<Object_DX>"
  Demux14/1 -> CAN FD Pack2/1
  Demux14/2 -> CAN FD Pack2/2
  Demux14/3 -> CAN FD Pack2/3
  Demux14/4 -> CAN FD Pack2/4
  Demux14/5 -> CAN FD Pack2/5
  Demux14/6 -> CAN FD Pack2/6
  Demux14/7 -> CAN FD Pack2/7
  Demux14/8 -> CAN FD Pack2/8
  Demux14/9 -> CAN FD Pack2/9
  Demux14/10 -> CAN FD Pack2/10
  Demux14/11 -> CAN FD Pack2/11
  Demux15/1 -> CAN FD Pack2/12
  Demux15/2 -> CAN FD Pack2/13
  Demux15/3 -> CAN FD Pack2/14
  Demux15/4 -> CAN FD Pack2/15
  Demux15/5 -> CAN FD Pack2/16
  Demux15/6 -> CAN FD Pack2/17
  Demux15/7 -> CAN FD Pack2/18
  Demux15/8 -> CAN FD Pack2/19
  Demux15/9 -> CAN FD Pack2/20
  Demux15/10 -> CAN FD Pack2/21
  Demux15/11 -> CAN FD Pack2/22
  Bus Selector/2 -> Demux15/1  "<Object_DY>"
  Bus Selector/4 -> Demux17/1  "<Object_Type>"
  Demux17/11 -> CAN FD Pack2/44
  Demux17/10 -> CAN FD Pack2/43
  Demux17/9 -> CAN FD Pack2/42
  Demux17/8 -> CAN FD Pack2/41
  Demux17/7 -> CAN FD Pack2/40
  Demux17/6 -> CAN FD Pack2/39
  Demux17/5 -> CAN FD Pack2/38
  Demux17/4 -> CAN FD Pack2/37
  Demux17/3 -> CAN FD Pack2/36
  Demux17/2 -> CAN FD Pack2/35
  Demux17/1 -> CAN FD Pack2/34
  Demux16/11 -> CAN FD Pack2/33
  Demux16/10 -> CAN FD Pack2/32
  Demux16/9 -> CAN FD Pack2/31
  Demux16/8 -> CAN FD Pack2/30
  Demux16/7 -> CAN FD Pack2/29
  Demux16/6 -> CAN FD Pack2/28
  Demux16/5 -> CAN FD Pack2/27
  Demux16/4 -> CAN FD Pack2/26
  Demux16/3 -> CAN FD Pack2/25
  Demux16/2 -> CAN FD Pack2/24
  Demux16/1 -> CAN FD Pack2/23
  Bus Selector/3 -> Demux16/1  "<Object_Fus_Type>"
  Bus Selector/5 -> Demux18/1  "<Object_VX>"
  Demux18/1 -> CAN FD Pack2/45
  Demux18/2 -> CAN FD Pack2/46
  Demux18/3 -> CAN FD Pack2/47
  Demux18/4 -> CAN FD Pack2/48
  Demux18/5 -> CAN FD Pack2/49
  Demux18/6 -> CAN FD Pack2/50
  Demux18/7 -> CAN FD Pack2/51
  Demux18/8 -> CAN FD Pack2/52
  Demux18/9 -> CAN FD Pack2/53
  Demux18/10 -> CAN FD Pack2/54
  Demux18/11 -> CAN FD Pack2/55
  CAN FD Pack2/1 -> TOS_LC1_Msg/1
  Demux19/1 -> CAN FD Pack3/1
  Demux19/2 -> CAN FD Pack3/2
  Demux19/3 -> CAN FD Pack3/3
  Demux19/4 -> CAN FD Pack3/4
  Demux19/5 -> CAN FD Pack3/5
  Demux19/6 -> CAN FD Pack3/6
  Demux19/7 -> CAN FD Pack3/7
  Demux19/8 -> CAN FD Pack3/8
  Demux19/9 -> CAN FD Pack3/9
  Demux19/10 -> CAN FD Pack3/10
  Demux19/11 -> CAN FD Pack3/11
  Demux20/11 -> CAN FD Pack3/22
  Demux20/10 -> CAN FD Pack3/21
  Demux20/9 -> CAN FD Pack3/20
  Demux20/8 -> CAN FD Pack3/19
  Demux20/7 -> CAN FD Pack3/18
  Demux20/6 -> CAN FD Pack3/17
  Demux20/5 -> CAN FD Pack3/16
  Demux20/4 -> CAN FD Pack3/15
  Demux20/3 -> CAN FD Pack3/14
  Demux20/2 -> CAN FD Pack3/13
  Demux20/1 -> CAN FD Pack3/12
  Demux22/1 -> CAN FD Pack3/34
  Demux22/2 -> CAN FD Pack3/35
  Demux22/3 -> CAN FD Pack3/36
  Demux22/4 -> CAN FD Pack3/37
  Demux22/5 -> CAN FD Pack3/38
  Demux22/6 -> CAN FD Pack3/39
  Demux22/7 -> CAN FD Pack3/40
  Demux22/8 -> CAN FD Pack3/41
  Demux22/9 -> CAN FD Pack3/42
  Demux22/10 -> CAN FD Pack3/43
  Demux22/11 -> CAN FD Pack3/44
  Demux21/11 -> CAN FD Pack3/33
  Demux21/10 -> CAN FD Pack3/32
  Demux21/9 -> CAN FD Pack3/31
  Demux21/8 -> CAN FD Pack3/30
  Demux21/7 -> CAN FD Pack3/29
  Demux21/6 -> CAN FD Pack3/28
  Demux21/5 -> CAN FD Pack3/27
  Demux21/4 -> CAN FD Pack3/26
  Demux21/3 -> CAN FD Pack3/25
  Demux21/2 -> CAN FD Pack3/24
  Demux21/1 -> CAN FD Pack3/23
  Demux23/1 -> CAN FD Pack3/45
  Demux23/2 -> CAN FD Pack3/46
  Demux23/3 -> CAN FD Pack3/47
  Demux23/4 -> CAN FD Pack3/48
  Demux23/5 -> CAN FD Pack3/49
  Demux23/6 -> CAN FD Pack3/50
  Demux23/7 -> CAN FD Pack3/51
  Demux23/8 -> CAN FD Pack3/52
  Demux23/9 -> CAN FD Pack3/53
  Demux23/10 -> CAN FD Pack3/54
  Demux23/11 -> CAN FD Pack3/55
  Demux24/1 -> CAN FD Pack3/56
  Demux24/2 -> CAN FD Pack3/57
  Demux24/3 -> CAN FD Pack3/58
  Demux24/4 -> CAN FD Pack3/59
  Demux24/5 -> CAN FD Pack3/60
  Demux24/6 -> CAN FD Pack3/61
  Demux24/7 -> CAN FD Pack3/62
  Demux24/8 -> CAN FD Pack3/63
  Demux24/9 -> CAN FD Pack3/64
  Demux24/10 -> CAN FD Pack3/65
  Demux24/11 -> CAN FD Pack3/66
  Bus Selector4/1 -> Demux19/1  "<CurrentLane_Prob>"
  Bus Selector4/6 -> Demux24/1  "<Object_ObstacleProb>"
  Bus Selector4/5 -> Demux23/1  "<Object_ID>"
  Bus Selector4/4 -> Demux22/1  "<Object_ExistProb>"
  Bus Selector4/3 -> Demux21/1  "<ObjectIn_Lane>"
  Bus Selector4/2 -> Demux20/1  "<LeftLane_Prob>"
  CAN FD Pack3/1 -> TOS_LC2_Msg/1
  Demux25/3 -> CAN FD Pack4/3
  Demux25/2 -> CAN FD Pack4/2
  Demux25/4 -> CAN FD Pack4/4
  Demux25/1 -> CAN FD Pack4/1
  Demux25/5 -> CAN FD Pack4/5
  Demux25/6 -> CAN FD Pack4/6
  Demux25/7 -> CAN FD Pack4/7
  Demux25/8 -> CAN FD Pack4/8
  Demux25/9 -> CAN FD Pack4/9
  Demux26/1 -> CAN FD Pack4/10
  Demux26/2 -> CAN FD Pack4/11
  Demux26/3 -> CAN FD Pack4/12
  Demux26/4 -> CAN FD Pack4/13
  Demux26/5 -> CAN FD Pack4/14
  Demux26/6 -> CAN FD Pack4/15
  Demux26/7 -> CAN FD Pack4/16
  Demux26/8 -> CAN FD Pack4/17
  Demux26/9 -> CAN FD Pack4/18
  Demux28/9 -> CAN FD Pack4/36
  Demux28/8 -> CAN FD Pack4/35
  Demux28/7 -> CAN FD Pack4/34
  Demux28/6 -> CAN FD Pack4/33
  Demux28/5 -> CAN FD Pack4/32
  Demux28/4 -> CAN FD Pack4/31
  Demux28/3 -> CAN FD Pack4/30
  Demux28/2 -> CAN FD Pack4/29
  Demux28/1 -> CAN FD Pack4/28
  Demux27/9 -> CAN FD Pack4/27
  Demux27/8 -> CAN FD Pack4/26
  Demux27/7 -> CAN FD Pack4/25
  Demux27/6 -> CAN FD Pack4/24
  Demux27/5 -> CAN FD Pack4/23
  Demux27/1 -> CAN FD Pack4/19
  Demux27/4 -> CAN FD Pack4/22
  Demux27/2 -> CAN FD Pack4/20
  Demux27/3 -> CAN FD Pack4/21
  Demux29/1 -> CAN FD Pack4/37
  Demux29/2 -> CAN FD Pack4/38
  Demux29/3 -> CAN FD Pack4/39
  Demux29/4 -> CAN FD Pack4/40
  Demux29/5 -> CAN FD Pack4/41
  Demux29/6 -> CAN FD Pack4/42
  Demux29/7 -> CAN FD Pack4/43
  Demux29/8 -> CAN FD Pack4/44
  Demux29/9 -> CAN FD Pack4/45
  Demux30/1 -> CAN FD Pack4/46
  Demux30/2 -> CAN FD Pack4/47
  Demux30/3 -> CAN FD Pack4/48
  Demux30/4 -> CAN FD Pack4/49
  Demux30/5 -> CAN FD Pack4/50
  Demux30/6 -> CAN FD Pack4/51
  Demux30/7 -> CAN FD Pack4/52
  Demux30/8 -> CAN FD Pack4/53
  Demux30/9 -> CAN FD Pack4/54
  Bus Selector1/1 -> Demux25/1  "<Object_DX>"
  Bus Selector1/2 -> Demux26/1  "<Object_DY>"
  Bus Selector1/3 -> Demux27/1  "<Object_ExistProb>"
  Bus Selector1/5 -> Demux29/1  "<Object_ID>"
  Bus Selector1/6 -> Demux30/1  "<Object_Type>"
  Bus Selector1/4 -> Demux28/1  "<Object_Fus_Type>"
  CAN FD Pack4/1 -> TOS_LCKie1_Msg/1
  Bus Selector5/4 -> Demux34/1  "<Object_VX>"
  Bus Selector5/5 -> Demux35/1  "<RightLane_Prob>"
  Bus Selector5/3 -> Demux33/1  "<ObjectIn_Lane>"
  Bus Selector5/2 -> Demux32/1  "<LeftLane_Prob>"
  Bus Selector5/1 -> Demux31/1  "<CurrentLane_Prob>"
  Demux35/9 -> CAN FD Pack5/45
  Demux35/8 -> CAN FD Pack5/44
  Demux35/7 -> CAN FD Pack5/43
  Demux35/6 -> CAN FD Pack5/42
  Demux35/5 -> CAN FD Pack5/41
  Demux35/4 -> CAN FD Pack5/40
  Demux35/3 -> CAN FD Pack5/39
  Demux35/2 -> CAN FD Pack5/38
  Demux35/1 -> CAN FD Pack5/37
  Demux33/3 -> CAN FD Pack5/21
  Demux33/2 -> CAN FD Pack5/20
  Demux33/4 -> CAN FD Pack5/22
  Demux33/1 -> CAN FD Pack5/19
  Demux33/5 -> CAN FD Pack5/23
  Demux33/6 -> CAN FD Pack5/24
  Demux33/7 -> CAN FD Pack5/25
  Demux33/8 -> CAN FD Pack5/26
  Demux33/9 -> CAN FD Pack5/27
  Demux34/1 -> CAN FD Pack5/28
  Demux34/2 -> CAN FD Pack5/29
  Demux34/3 -> CAN FD Pack5/30
  Demux34/4 -> CAN FD Pack5/31
  Demux34/5 -> CAN FD Pack5/32
  Demux34/6 -> CAN FD Pack5/33
  Demux34/7 -> CAN FD Pack5/34
  Demux34/8 -> CAN FD Pack5/35
  Demux34/9 -> CAN FD Pack5/36
  Demux32/9 -> CAN FD Pack5/18
  Demux32/8 -> CAN FD Pack5/17
  Demux32/7 -> CAN FD Pack5/16
  Demux32/6 -> CAN FD Pack5/15
  Demux32/5 -> CAN FD Pack5/14
  Demux32/4 -> CAN FD Pack5/13
  Demux32/3 -> CAN FD Pack5/12
  Demux32/2 -> CAN FD Pack5/11
  Demux32/1 -> CAN FD Pack5/10
  Demux31/9 -> CAN FD Pack5/9
  Demux31/8 -> CAN FD Pack5/8
  Demux31/7 -> CAN FD Pack5/7
  Demux31/6 -> CAN FD Pack5/6
  Demux31/5 -> CAN FD Pack5/5
  Demux31/1 -> CAN FD Pack5/1
  Demux31/4 -> CAN FD Pack5/4
  Demux31/2 -> CAN FD Pack5/2
  Demux31/3 -> CAN FD Pack5/3
  TOS_LCKIE/1 -> Bus Selector5/1, Bus Selector1/1
  CAN FD Pack5/1 -> TOS_LCKie2_Msg/1

== system PubIfDecisionTOS_MDL/TOS_20201112/TOS_2012080320/TLJ ==
  TOS_AddAttributes : Inport
  OFM_SignalVerification : Inport  Port=2
  PIL_ProbInLaneCalculat : Inport  Port=3
  Bus Creator : BusCreator  Inputs=3
  Bus Creator1 : BusCreator  Inputs=4
  Bus Selector : BusSelector  OutputSignals=OFM_SignalVerification.TOS_OFMObjValid_Flag,PIL_ProbInLaneCalculat.PIL_ObjLaneProb_all,PIL_ProbInLaneCalculat.PIL_CurrentLaneProb,PIL_ProbInLaneCalculat.PIL_LeftLaneProb,PIL_ProbInLaneCalculat.PIL_RightLaneProb,PIL_ProbInLaneCalculat.TOS_PIL_EgoVehiclePro.EgoCar_CurrentLaneProb,PIL_ProbInLaneCalculat.TOS_PIL_EgoVehiclePro.EgoCar_LeftLaneProb,PIL_ProbInLaneCalculat.TOS_PIL_EgoVehiclePro.EgoCar_RightLaneProb,OFM_SignalVerification.Object_Type,OFM_SignalVerification.Object_DY,PIL_ProbInLaneCalculat.PIL_CutinFlag,PIL_ProbInLaneCalculat.PIL_CutoutFlag
  Pro : Subsystem
  Terminator3 : Terminator
  TLJ_LeftLaneConfirm_Flag : Outport
  TLJ_SameLaneConfirm_Flag : Outport  Port=2
  TLJ_RightLaneConfirm_Flag : Outport  Port=3
  wires:
  Bus Creator/1 -> Bus Selector/1
  TOS_AddAttributes/1 -> Bus Creator/1
  OFM_SignalVerification/1 -> Bus Creator/2
  PIL_ProbInLaneCalculat/1 -> Bus Creator/3
  Bus Selector/1 -> Pro/1(TOS_OFMObjValid_Flag)  "<TOS_OFMObjValid_Flag>"
  Pro/2(TLJ_ObjInEgoLane_flag) -> TLJ_SameLaneConfirm_Flag/1  "TOS_TLJ_SameLaneConfirm_Flag"
  Pro/1(TLJ_ObjInLeftLane_flag) -> TLJ_LeftLaneConfirm_Flag/1  "TOS_TLJ_LeftLaneConfirm_Flag"
  Pro/3(TLJ_ObjInRightLane_flag) -> TLJ_RightLaneConfirm_Flag/1  "TOS_TLJ_RightLaneConfirm_Flag"
  Bus Selector/2 -> Pro/2(PIL_ObjLaneProb_all)  "<PIL_ObjLaneProb_all>"
  Bus Selector/3 -> Pro/3(PIL_EgoLaneProb)  "<PIL_CurrentLaneProb>"
  Bus Selector/4 -> Pro/4(PIL_LeftLaneProb)  "<PIL_LeftLaneProb>"
  Bus Selector/5 -> Pro/5(PIL_RightLaneProb)  "<PIL_RightLaneProb>"
  Bus Selector/6 -> Pro/6(PIL_EgoVehicle_EgoLaneProb)  "<EgoCar_CurrentLaneProb>"
  Bus Selector/7 -> Pro/7(PIL_EgoVehicle_LeftLaneProb)  "<EgoCar_LeftLaneProb>"
  Bus Selector/8 -> Pro/8(PIL_EgoVehicle_RightLaneProb)  "<EgoCar_RightLaneProb>"
  Bus Selector/9 -> Pro/9(Object_Type)  "<Object_Type>"
  Bus Selector/11 -> Pro/11(PIL_CutinFlag)  "<PIL_CutinFlag>"
  Pro/4(TOS_TLJ_ObjinLeftLaneProb_ObserVale) -> Bus Creator1/1  "TOS_TLJ_ObjinLeftLaneProb_ObserVale"
  Pro/5(TOS_TLJ_ObjinEgoLaneProb_ObserVale) -> Bus Creator1/2  "TOS_TLJ_ObjinEgoLaneProb_ObserVale"
  Pro/6(TOS_TLJ_ObjinRightLaneProb_ObserVale) -> Bus Creator1/3  "TOS_TLJ_ObjinRightLaneProb_ObserVale"
  Pro/7(TOS_TLJ_ObjInLaneCondition_Flag_ObserVale) -> Bus Creator1/4  "TOS_TLJ_ObjInLaneCondition_Flag_ObserVale"
  Bus Selector/10 -> Pro/10(Object_DY)  "<Object_DY>"
  Bus Selector/12 -> Pro/12(PIL_CutoutFlag)  "<PIL_CutoutFlag>"
  Bus Creator1/1 -> Terminator3/1  "TOS_TLJ_ObserVale"
